simulink model "schemat"  (R2021b)
settings: Solver=VariableStepAuto  StartTime=0.0  StopTime=10.0  RelTol=1e-3
values from neighbouring files (symbols this model uses):
  I = 2    [lab4.m]
  Kz = c2d(K,Ts,'foh')    [lab4.m]
  Kz1 = c2d(K1,Ts,'foh')    [lab4.m]
  Kz2 = c2d(K2,Ts,'foh')    [lab4.m]
  P = 6    [lab4.m]
  Ts = i    [lab4.m]
libraries: slpidlib x1
settings Model: Creator=pc  LastModifiedBy=pc
settings DebuggingCC: AlgebraicLoopMsg=none

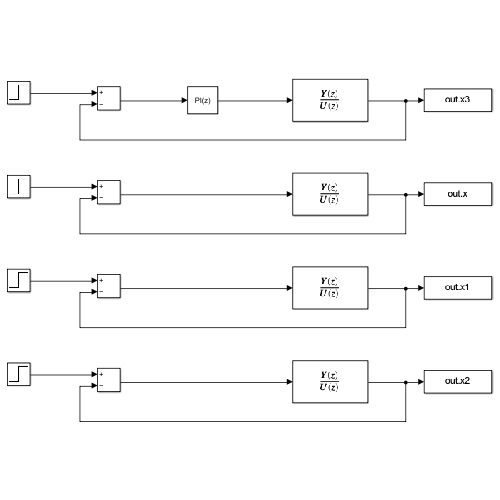
[thumbnail: Simulink's stored preview of the top-level diagram]
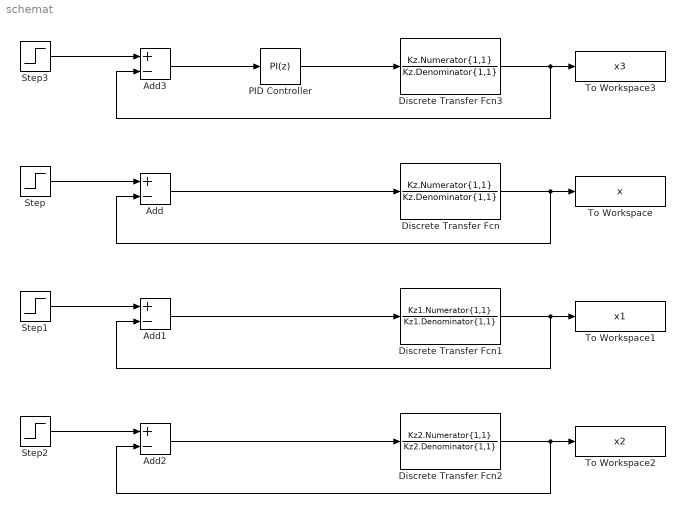
== system schemat ==
  Add{,1..3} (4 alike) : Sum  Inputs=+-
  Discrete Transfer Fcn : DiscreteTransferFcn  Numerator=Kz.Numerator{1,1}  Denominator=Kz.Denominator{1,1}
  Discrete Transfer Fcn1 : DiscreteTransferFcn  Numerator=Kz1.Numerator{1,1}  Denominator=Kz1.Denominator{1,1}
  Discrete Transfer Fcn2 : DiscreteTransferFcn  Numerator=Kz2.Numerator{1,1}  Denominator=Kz2.Denominator{1,1}
  Discrete Transfer Fcn3 : DiscreteTransferFcn  Numerator=Kz.Numerator{1,1}  Denominator=Kz.Denominator{1,1}
  PID Controller : slpidlib/PID Controller  Controller=PI  Form=Parallel  TimeDomain=Discrete-time  UseExternalTs=off  SampleTime=Ts  IntegratorMethod=Forward Euler  FilterMethod=Forward Euler  ControllerParametersSource=internal  P=P  I=I  D=0  UseFilter=on  N=100  TunerSelectOption=Transfer Function Based (PID Tuner App)  InitialConditionSource=internal  InitialConditionForIntegrator=0  InitialConditionForFilter=0  DifferentiatorICPrevScaledInput=0  ExternalReset=none  TrackingMode=off  Kt=1  LimitOutput=off  SatLimitsSource=internal  UpperSaturationLimit=inf  LowerSaturationLimit=-inf  LinearizeAsGain=on  AntiWindupMode=none  Kb=1  POutMin=[]  POutMax=[]  IOutMin=[]  IOutMax=[]  DOutMin=[]  DOutMax=[]  NOutMin=[]  NOutMax=[]  SumOutMin=[]  SumOutMax=[]  SaturationOutMin=[]  SaturationOutMax=[]  PParamMin=[]  PParamMax=[]  IParamMin=[]  IParamMax=[]  DParamMin=[]  DParamMax=[]  NParamMin=[]  NParamMax=[]  KbParamMin=[]  KbParamMax=[]  KtParamMin=[]  KtParamMax=[]  KbOutMin=[]  KbOutMax=[]  KtOutMin=[]  KtOutMax=[]  IntegratorOutMin=[]  IntegratorOutMax=[]  FilterOutMin=[]  FilterOutMax=[]  SumI1OutMin=[]  SumI1OutMax=[]  SumI2OutMin=[]  SumI2OutMax=[]  SumI3OutMin=[]  SumI3OutMax=[]  SumI4OutMin=[]  SumI4OutMax=[]  SumDOutMin=[]  SumDOutMax=[]  DifferentiatorOutMin=[]  DifferentiatorOutMax=[]  FilterDiffOutCoefMin=[]  FilterDiffOutCoefMax=[]  ReciprocalOutMin=[]  ReciprocalOutMax=[]  SumDenOutMin=[]  SumDenOutMax=[]  SumNumOutMin=[]  SumNumOutMax=[]  DivideOutMin=[]  DivideOutMax=[]  UdiffTsProdOutMin=[]  UdiffTsProdOutMax=[]  NTsProdOutMin=[]  NTsProdOutMax=[]  UintegralTsProdOutMin=[]  UintegralTsProdOutMax=[]  UngainTsProdOutMin=[]  UngainTsProdOutMax=[]  IntegratorContinuousStateAttributes=''  IntegratorStateMustResolveToSignalObject=off  IntegratorRTWStateStorageClass=Auto  FilterContinuousStateAttributes=''  FilterStateMustResolveToSignalObject=off  FilterRTWStateStorageClass=Auto  ParallelPVariant=InternalParameters  IdealPVariant=Disabled  IVariant=InternalParameters  DVariant=Disabled  IntegratorVariant=Discrete  SatVariant=Disabled  AWVariant=Passthrough  PCopyVariant=Disabled  TRVariant=Disabled  FdbkBlocksVariant=Forward  IdealPFdbkVariant=Disabled  SatFdbkVariant=Disabled  DerivativeFilterVariant=Disabled  NVariant=Disabled  NCopyVariant=Disabled_SignalSpec  FilterICVariant=Disabled  IntegratorICVariant=InternalICs  ExternalResetVariant=Disabled  TRSumVariant=Passthrough  SumFdbkVariant=Disabled  SumVariant=Sum_PI  TsampFilterVariant=InternalTs  TsampNgainVariant=Passthrough  TsampIntegralVariant=Passthrough  ExternalSaturationOutDataTypeStr=Inherit: Same as second input
  Step{,1..3} (4 alike) : Step  SampleTime=0  ZeroCross=off
  To Workspace : ToWorkspace  VariableName=x  SampleTime=-1
  To Workspace1 : ToWorkspace  VariableName=x1  SampleTime=-1
  To Workspace2 : ToWorkspace  VariableName=x2  SampleTime=-1
  To Workspace3 : ToWorkspace  VariableName=x3  SampleTime=-1
  wires:
  Step/1 -> Add/1
  Discrete Transfer Fcn/1 -> Add/2, To Workspace/1
  Add/1 -> Discrete Transfer Fcn/1
  Add1/1 -> Discrete Transfer Fcn1/1
  Discrete Transfer Fcn1/1 -> Add1/2, To Workspace1/1
  Step1/1 -> Add1/1
  Add2/1 -> Discrete Transfer Fcn2/1
  Discrete Transfer Fcn2/1 -> Add2/2, To Workspace2/1
  Step2/1 -> Add2/1
  Discrete Transfer Fcn3/1 -> Add3/2, To Workspace3/1
  Step3/1 -> Add3/1
  Add3/1 -> PID Controller/1
  PID Controller/1 -> Discrete Transfer Fcn3/1
